simulink model "RefModel_GroundStation_FlightData"  (R2020b)
settings: Solver=FixedStepAuto  StartTime=0.0  StopTime=150  FixedStep=SimParam.GroundStation.Ts_base  RelTol=1e-3
values from neighbouring files (symbols this model uses):
  TASK_PARAM_V1000 = Simulink.Bus.createMATLABStruct('BUS_TASK_PATH_AlgoParam')    [INIT_Task.m]    (also in INIT_TaskManage.m)
undefined symbols (not defined in the file or in its folder): count, distBack, distFront, distLeft, distRight, ENUM_FlightTaskMode, flightTaskMode, groundspeedCmd, headingCmd, heightCmd, isRemoteConnected, isStationConnected, maxClimbSpeed, nBack, nFront, nLeft, nRight, param1_lond, param1_pointNumber, param2_latd, param3_relativeHeight, param4_radius, SimParam, stationLostTimeSec, unlock
settings Model: PauseTimes=0  Creator=sl  LastModifiedBy=sl
settings DataIOCC: SaveOutput=off  SaveTime=off  ReturnWorkspaceOutputs=off
settings DebuggingCC: InheritedTsInSrcMsg=none  UnderSpecifiedDimensionMsg=warning  ArithmeticOperatorsInVariantConditions=warning
settings SFSimCC: CustomCodeUndefinedFunction=UseInterfaceOnly
settings GRTTargetCC: CombineOutputUpdateFcns=off  MatFileLogging=off

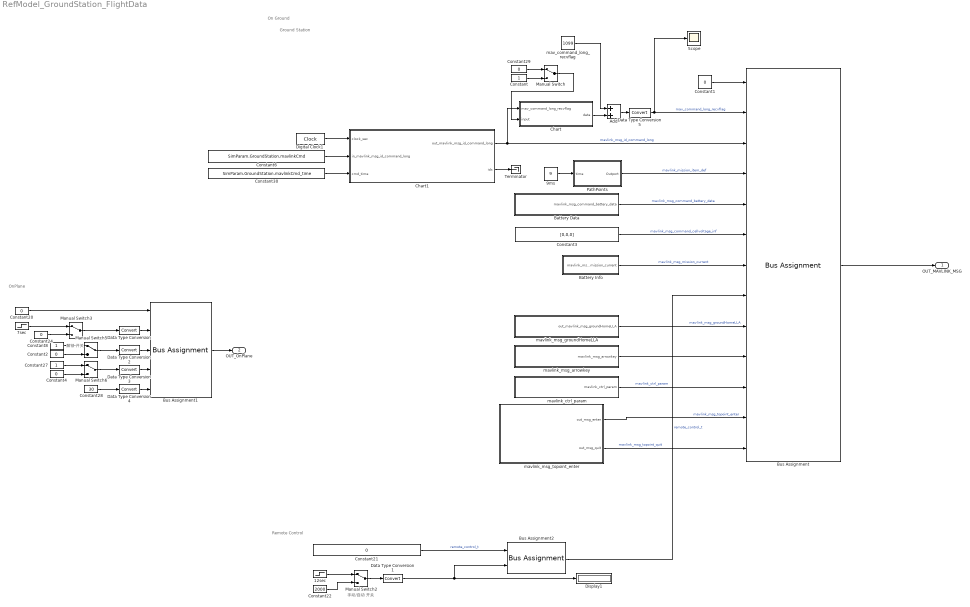
== system RefModel_GroundStation_FlightData ==
  note: 手动/自动 开关
  note: Ground Station
  note: Remote Control
  note: OnPlane
  note: On Ground
  note: 解锁 开关
  12sec : Step  Time=12+30  Before=2000  After=1000  SampleTime=SimParam.GroundStation.Ts_base  mask(DiscretizedSource){}
      mask init:
      | %zoh
  7sec : Step  Time=7+30  SampleTime=SimParam.GroundStation.Ts_base  mask(DiscretizedSource){}
      mask init:
      | %zoh
  9ms : Constant  Value=9
  Add : Sum
  Battery Data : Subsystem
  Battery Info : Subsystem
  Bus Assignment : BusAssignment  AssignedSignals=mav_command_long_recvflag,mavlink_msg_id_command_long,mavlink_mission_item_def,mavlink_msg_command_battery_data,mavlink_msg_command_cellvoltage_inf,mavlink_msg_mission_current,remote_control_t,mavlink_msg_groundHomeLLA,mavlink_msg_arrowkey,mavlink_ctrl_param,mavlink_msg_topoint_enter,mavlink_msg_topoint_quit
  Bus Assignment1 : BusAssignment  AssignedSignals=unlock,isRemoteConnected,isStationConnected,stationLostTimeSec
  Bus Assignment2 : BusAssignment  AssignedSignals=chG_Mag
  Chart : Stateflow chart  TreatAsAtomicUnit=on
  Chart1 : Stateflow chart  TreatAsAtomicUnit=on
  Constant : Constant
  Constant1 : Constant  Value=0  OutDataTypeStr=Bus: BUS_MAVLINK_TO_FIRM
  Constant{2,4,24,29} (4 alike) : Constant  Value=0
  Constant20 : Constant  Value=0  OutDataTypeStr=Bus: BUS_ONPLANE_FEEDBACK
  Constant21 : Constant  Value=0  OutDataTypeStr=Bus: remote_control_t
  Constant22 : Constant  Value=2000
  Constant27 : Constant
  Constant28 : Constant  Value=30
  Constant3 : Constant  Value=[0,0,0]  OutDataTypeStr=Bus: mavlink_msg_command_cellvoltage_inf
  Constant30 : Constant  Value=SimParam.GroundStation.mavlinkCmd_time
  Constant6 : Constant  Value=SimParam.GroundStation.mavlinkCmd  OutDataTypeStr=Bus: mavlink_msg_id_command_long
  Constant8 : Constant
  Data Type Conversion{,1..5} (6 alike) : DataTypeConversion
  Digital Clock1 : DigitalClock  SampleTime=-1
  Display1 : Display
  Manual Switch{,2..3,5..6} (5 alike) : ManualSwitch
  PathPoints : Subsystem
  Scope : Scope
  Terminator : Terminator
  mav_command_long_recvflag : Constant  Value=1099
  mavlink_ctrl_param : Subsystem
  mavlink_msg_arrowkey : Subsystem
  mavlink_msg_groundHomeLLA : Subsystem
  mavlink_msg_topoint_enter : Subsystem
  OUT_MAVLINK_MSG : Outport  OutDataTypeStr=Bus: BUS_MAVLINK_TO_FIRM  BusOutputAsStruct=on
  OUT_OnPlane : Outport  Port=2  OutDataTypeStr=Bus: BUS_ONPLANE_FEEDBACK
  wires:
  Bus Assignment/1 -> OUT_MAVLINK_MSG/1
  Bus Assignment1/1 -> OUT_OnPlane/1
  Battery Info/1(mavlink_msg_mission_current) -> Bus Assignment/7  "mavlink_msg_mission_current"
  Constant3/1 -> Bus Assignment/6  "mavlink_msg_command_cellvoltage_inf"
  PathPoints/1(Outport) -> Bus Assignment/4  "mavlink_mission_item_def"
  Chart1/1(out_mavlink_msg_id_command_long) -> Bus Assignment/3, Chart/1(mav_command_long_recvflag)  "mavlink_msg_id_command_long"
  Constant20/1 -> Bus Assignment1/1
  Constant21/1 -> Bus Assignment2/1  "remote_control_t"
  Bus Assignment2/1 -> Bus Assignment/8  "remote_control_t"
  Data Type Conversion1/1 -> Bus Assignment2/2, Display1/1
  Manual Switch2/1 -> Data Type Conversion1/1
  12sec/1 -> Manual Switch2/1
  Constant22/1 -> Manual Switch2/2
  Constant24/1 -> Manual Switch3/2
  Data Type Conversion/1 -> Bus Assignment1/2
  7sec/1 -> Manual Switch3/1
  Manual Switch3/1 -> Data Type Conversion/1
  Battery Data/1(mavlink_msg_command_battery_data) -> Bus Assignment/5  "mavlink_msg_command_battery_data"
  Data Type Conversion2/1 -> Bus Assignment1/3
  Data Type Conversion3/1 -> Bus Assignment1/4
  Data Type Conversion4/1 -> Bus Assignment1/5
  Constant28/1 -> Data Type Conversion4/1
  Manual Switch5/1 -> Data Type Conversion2/1
  Constant8/1 -> Manual Switch5/1
  Constant2/1 -> Manual Switch5/2
  Constant4/1 -> Manual Switch6/2
  Constant27/1 -> Manual Switch6/1
  Manual Switch6/1 -> Data Type Conversion3/1
  9ms/1 -> PathPoints/1(time)
  Constant29/1 -> Manual Switch/1
  Constant/1 -> Manual Switch/2
  Manual Switch/1 -> Chart/2(input)
  Data Type Conversion5/1 -> Bus Assignment/2, Scope/1  "mav_command_long_recvflag"
  mavlink_msg_groundHomeLLA/1(out_mavlink_msg_groundHomeLLA) -> Bus Assignment/9  "mavlink_msg_groundHomeLLA"
  Chart/1(data) -> Add/2
  Add/1 -> Data Type Conversion5/1
  mav_command_long_recvflag/1 -> Add/1
  mavlink_msg_arrowkey/1(mavlink_msg_arrowkey) -> Bus Assignment/10
  mavlink_ctrl_param/1(mavlink_ctrl_param) -> Bus Assignment/11  "mavlink_ctrl_param"
  Constant30/1 -> Chart1/3(cmd_time)
  Digital Clock1/1 -> Chart1/1(clock_sec)
  Constant6/1 -> Chart1/2(in_mavlink_msg_id_command_long)
  Chart1/2(idx) -> Terminator/1
  mavlink_msg_topoint_enter/2(out_msg_quit) -> Bus Assignment/13  "mavlink_msg_topoint_quit"
  mavlink_msg_topoint_enter/1(out_msg_enter) -> Bus Assignment/12  "mavlink_msg_topoint_enter"
  Constant1/1 -> Bus Assignment/1

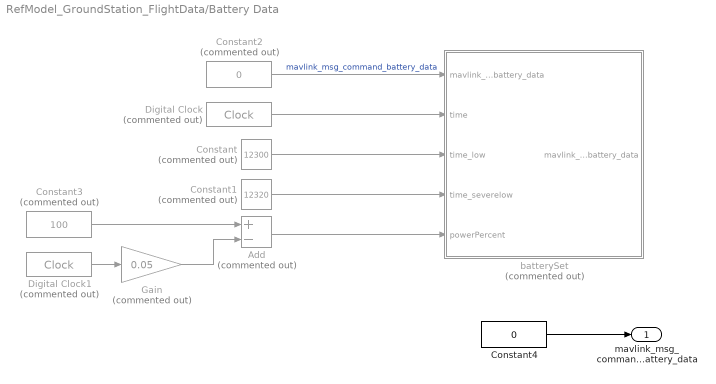
== system RefModel_GroundStation_FlightData/Battery Data ==
  Add : Sum  Commented=on  Inputs=+-
  Constant : Constant  Commented=on  Value=12300
  Constant1 : Constant  Commented=on  Value=12320
  Constant2 : Constant  Commented=on  Value=0  OutDataTypeStr=Bus: mavlink_msg_command_battery_data
  Constant3 : Constant  Commented=on  Value=100
  Constant4 : Constant  Value=0  OutDataTypeStr=Bus: mavlink_msg_command_battery_data
  Digital Clock : DigitalClock  Commented=on  SampleTime=-1
  Digital Clock1 : DigitalClock  Commented=on  SampleTime=-1
  Gain : Gain  Commented=on  Gain=0.05
  batterySet : MATLAB Function  Commented=on  TreatAsAtomicUnit=on
  mavlink_msg_command_battery_data : Outport
  wires:
  Constant2/1 -> batterySet/1("mavlink_msg_command_battery_data ")  "mavlink_msg_command_battery_data"
  Constant4/1 -> mavlink_msg_command_battery_data/1
  Digital Clock/1 -> batterySet/2(time)
  Constant/1 -> batterySet/3(time_low)
  Constant1/1 -> batterySet/4(time_severelow)
  Add/1 -> batterySet/5(powerPercent)
  Constant3/1 -> Add/1
  Digital Clock1/1 -> Gain/1
  Gain/1 -> Add/2

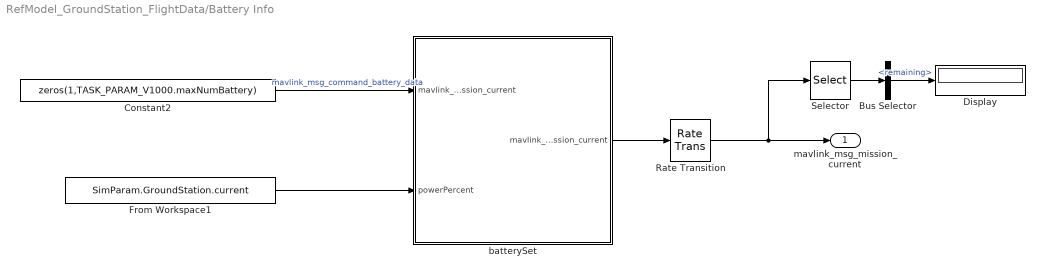
== system RefModel_GroundStation_FlightData/Battery Info ==
  Bus Selector : BusSelector  OutputSignals=remaining
  Constant2 : Constant  Value=zeros(1,TASK_PARAM_V1000.maxNumBattery)  OutDataTypeStr=Bus: mavlink_msg_mission_current
  Display : Display
  From Workspace1 : FromWorkspace  VariableName=SimParam.GroundStation.current  OutputAfterFinalValue=Holding final value
  Rate Transition : RateTransition
  Selector : Selector  InputPortWidth=TASK_PARAM_V1000.maxNumBattery  IndexOptions=Index vector (dialog)  Indices=1  OutputSizes=1
  batterySet : MATLAB Function  TreatAsAtomicUnit=on
  mavlink_msg_mission_current : Outport
  wires:
  From Workspace1/1 -> batterySet/2(powerPercent)
  batterySet/1(mavlink_msg_mission_current) -> Rate Transition/1
  Constant2/1 -> batterySet/1("mavlink_msg_mission_current ")  "mavlink_msg_command_battery_data"
  Rate Transition/1 -> Selector/1, mavlink_msg_mission_current/1
  Selector/1 -> Bus Selector/1
  Bus Selector/1 -> Display/1  "<remaining>"

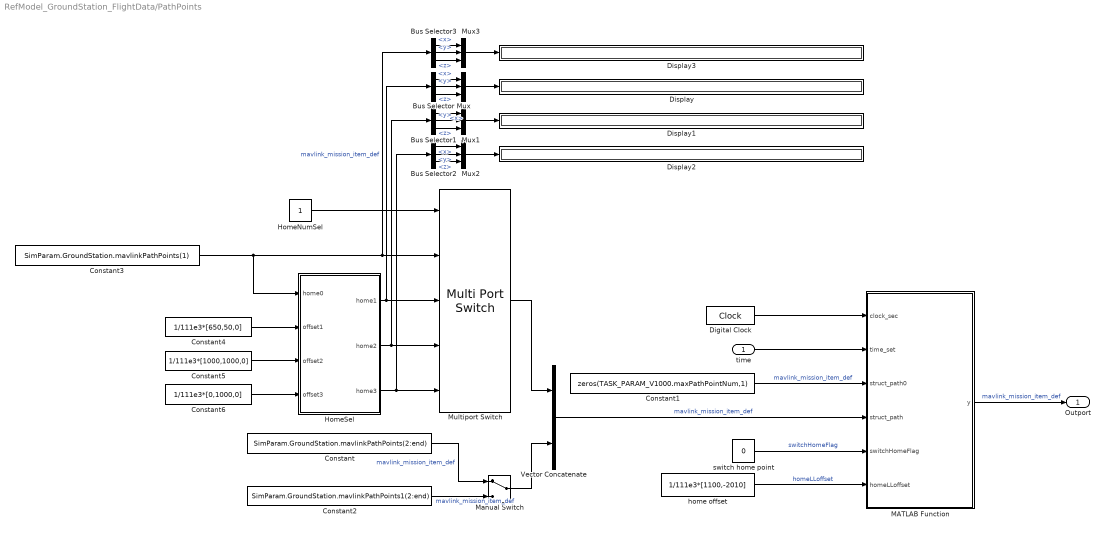
== system RefModel_GroundStation_FlightData/PathPoints ==
  time : Inport
  Bus Selector{,1..3} (4 alike) : BusSelector  OutputSignals=x,y,z
  Constant : Constant  Value=SimParam.GroundStation.mavlinkPathPoints(2:end)  OutDataTypeStr=Bus: mavlink_mission_item_def
  Constant1 : Constant  Value=zeros(TASK_PARAM_V1000.maxPathPointNum,1)  OutDataTypeStr=Bus: mavlink_mission_item_def
  Constant2 : Constant  Value=SimParam.GroundStation.mavlinkPathPoints1(2:end)  OutDataTypeStr=Bus: mavlink_mission_item_def
  Constant3 : Constant  Value=SimParam.GroundStation.mavlinkPathPoints(1)  OutDataTypeStr=Bus: mavlink_mission_item_def
  Constant4 : Constant  Value=1/111e3*[650,50,0]
  Constant5 : Constant  Value=1/111e3*[1000,1000,0]
  Constant6 : Constant  Value=1/111e3*[0,1000,0]
  Digital Clock : DigitalClock  SampleTime=-1
  Display{,1..3} (4 alike) : Display
  HomeNumSel : Constant
  HomeSel : MATLAB Function  TreatAsAtomicUnit=on
  MATLAB Function : MATLAB Function  TreatAsAtomicUnit=on
  Manual Switch : ManualSwitch
  Multiport Switch : MultiPortSwitch  Inputs=4
  Mux{,1..3} (4 alike) : Mux  Inputs=3
  Vector Concatenate : Concatenate
  home offset : Constant  Value=1/111e3*[1100,-2010]
  switch home point : Constant  Value=0
  Outport : Outport
  wires:
  MATLAB Function/1(y) -> Outport/1  "mavlink_mission_item_def"
  Digital Clock/1 -> MATLAB Function/1(clock_sec)
  time/1 -> MATLAB Function/2(time_set)
  Constant1/1 -> MATLAB Function/3(struct_path0)  "mavlink_mission_item_def"
  Vector Concatenate/1 -> MATLAB Function/4(struct_path)  "mavlink_mission_item_def"
  switch home point/1 -> MATLAB Function/5(switchHomeFlag)  "switchHomeFlag"
  home offset/1 -> MATLAB Function/6(homeLLoffset)  "homeLLoffset"
  Constant/1 -> Manual Switch/1  "mavlink_mission_item_def"
  HomeNumSel/1 -> Multiport Switch/1
  Multiport Switch/1 -> Vector Concatenate/1
  Constant3/1 -> HomeSel/1(home0), Bus Selector3/1, Multiport Switch/2  "mavlink_mission_item_def"
  Constant4/1 -> HomeSel/2(offset1)
  Constant5/1 -> HomeSel/3(offset2)
  Constant6/1 -> HomeSel/4(offset3)
  HomeSel/3(home3) -> Bus Selector2/1, Multiport Switch/5
  HomeSel/2(home2) -> Bus Selector1/1, Multiport Switch/4
  HomeSel/1(home1) -> Bus Selector/1, Multiport Switch/3
  Bus Selector/1 -> Mux/1  "<x>"
  Bus Selector/2 -> Mux/2  "<y>"
  Bus Selector/3 -> Mux/3  "<z>"
  Mux/1 -> Display/1
  Mux1/1 -> Display1/1
  Bus Selector1/3 -> Mux1/3  "<z>"
  Bus Selector1/2 -> Mux1/2  "<y>"
  Bus Selector1/1 -> Mux1/1  "<x>"
  Bus Selector2/1 -> Mux2/1  "<x>"
  Bus Selector2/2 -> Mux2/2  "<y>"
  Bus Selector2/3 -> Mux2/3  "<z>"
  Mux2/1 -> Display2/1
  Mux3/1 -> Display3/1
  Bus Selector3/3 -> Mux3/3  "<z>"
  Bus Selector3/2 -> Mux3/2  "<y>"
  Bus Selector3/1 -> Mux3/1  "<x>"
  Constant2/1 -> Manual Switch/2  "mavlink_mission_item_def"
  Manual Switch/1 -> Vector Concatenate/2

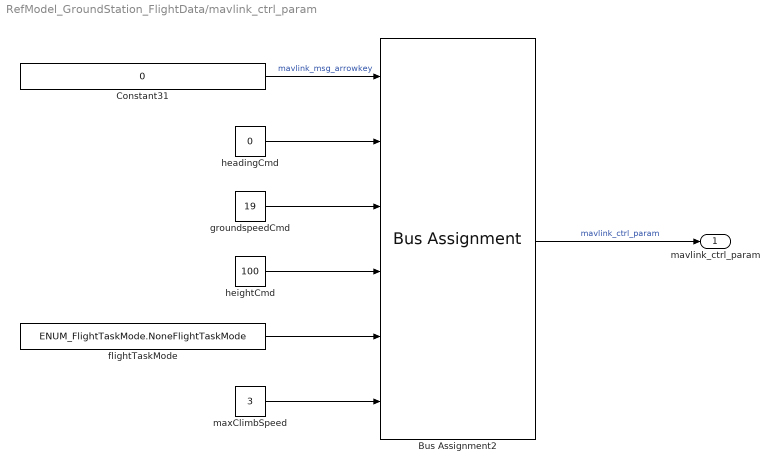
== system RefModel_GroundStation_FlightData/mavlink_ctrl_param ==
  Bus Assignment2 : BusAssignment  AssignedSignals=headingCmd,groundspeedCmd,heightCmd,flightTaskMode,maxClimbSpeed
  Constant31 : Constant  Value=0  OutDataTypeStr=Bus: mavlink_ctrl_param
  flightTaskMode : Constant  Value=ENUM_FlightTaskMode.NoneFlightTaskMode
  groundspeedCmd : Constant  Value=19
  headingCmd : Constant  Value=0
  heightCmd : Constant  Value=100
  maxClimbSpeed : Constant  Value=3
  mavlink_ctrl_param : Outport
  wires:
  Constant31/1 -> Bus Assignment2/1  "mavlink_msg_arrowkey"
  Bus Assignment2/1 -> mavlink_ctrl_param/1  "mavlink_ctrl_param"
  headingCmd/1 -> Bus Assignment2/2
  groundspeedCmd/1 -> Bus Assignment2/3
  heightCmd/1 -> Bus Assignment2/4
  maxClimbSpeed/1 -> Bus Assignment2/6
  flightTaskMode/1 -> Bus Assignment2/5

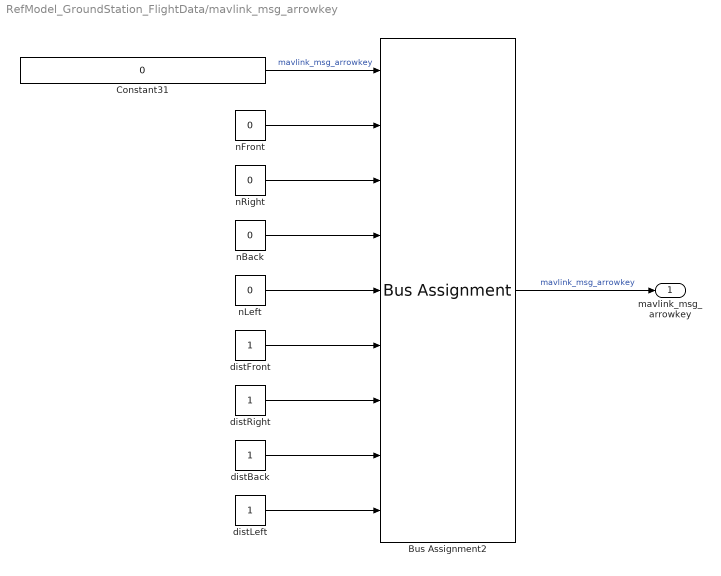
== system RefModel_GroundStation_FlightData/mavlink_msg_arrowkey ==
  Bus Assignment2 : BusAssignment  AssignedSignals=nFront,nRight,nBack,nLeft,distFront,distRight,distBack,distLeft
  Constant31 : Constant  Value=0  OutDataTypeStr=Bus: BUS_TASK_ARROWKEY
  distBack : Constant
  distFront : Constant
  distLeft : Constant
  distRight : Constant
  nBack : Constant  Value=0
  nFront : Constant  Value=0
  nLeft : Constant  Value=0
  nRight : Constant  Value=0
  mavlink_msg_arrowkey : Outport
  wires:
  Bus Assignment2/1 -> mavlink_msg_arrowkey/1  "mavlink_msg_arrowkey"
  Constant31/1 -> Bus Assignment2/1  "mavlink_msg_arrowkey"
  nFront/1 -> Bus Assignment2/2
  nRight/1 -> Bus Assignment2/3
  nBack/1 -> Bus Assignment2/4
  nLeft/1 -> Bus Assignment2/5
  distFront/1 -> Bus Assignment2/6
  distRight/1 -> Bus Assignment2/7
  distBack/1 -> Bus Assignment2/8
  distLeft/1 -> Bus Assignment2/9

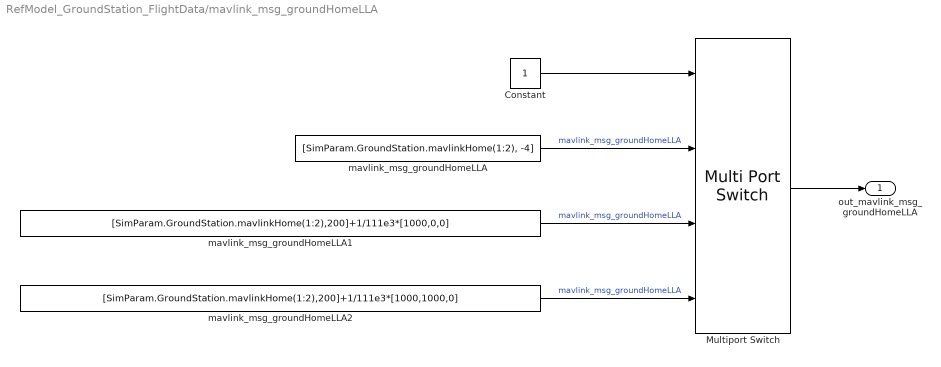
== system RefModel_GroundStation_FlightData/mavlink_msg_groundHomeLLA ==
  Constant : Constant
  Multiport Switch : MultiPortSwitch
  mavlink_msg_groundHomeLLA : Constant  Value=[SimParam.GroundStation.mavlinkHome(1:2), -4]  OutDataTypeStr=Inherit: Inherit via back propagation
  mavlink_msg_groundHomeLLA1 : Constant  Value=[SimParam.GroundStation.mavlinkHome(1:2),200]+1/111e3*[1000,0,0]  OutDataTypeStr=Inherit: Inherit via back propagation
  mavlink_msg_groundHomeLLA2 : Constant  Value=[SimParam.GroundStation.mavlinkHome(1:2),200]+1/111e3*[1000,1000,0]  OutDataTypeStr=Inherit: Inherit via back propagation
  out_mavlink_msg_groundHomeLLA : Outport
  wires:
  mavlink_msg_groundHomeLLA/1 -> Multiport Switch/2  "mavlink_msg_groundHomeLLA"
  Multiport Switch/1 -> out_mavlink_msg_groundHomeLLA/1
  Constant/1 -> Multiport Switch/1
  mavlink_msg_groundHomeLLA1/1 -> Multiport Switch/3  "mavlink_msg_groundHomeLLA"
  mavlink_msg_groundHomeLLA2/1 -> Multiport Switch/4  "mavlink_msg_groundHomeLLA"

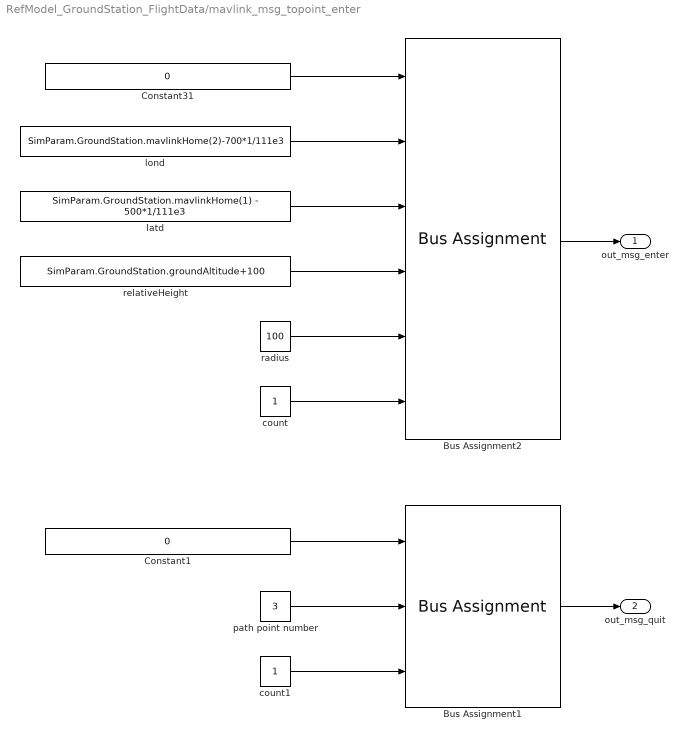
== system RefModel_GroundStation_FlightData/mavlink_msg_topoint_enter ==
  Bus Assignment1 : BusAssignment  AssignedSignals=param1_pointNumber,count
  Bus Assignment2 : BusAssignment  AssignedSignals=param1_lond,param2_latd,param3_relativeHeight,param4_radius,count
  Constant1 : Constant  Value=0  OutDataTypeStr=Bus: BUS_MAVLINK_ToPointAndHover_Quit
  Constant31 : Constant  Value=0  OutDataTypeStr=Bus: BUS_MAVLINK_ToPointAndHover_Enter
  count : Constant
  count1 : Constant
  latd : Constant  Value=SimParam.GroundStation.mavlinkHome(1) - 500*1/111e3
  lond : Constant  Value=SimParam.GroundStation.mavlinkHome(2)-700*1/111e3
  path point number : Constant  Value=3
  radius : Constant  Value=100
  relativeHeight : Constant  Value=SimParam.GroundStation.groundAltitude+100
  out_msg_enter : Outport
  out_msg_quit : Outport  Port=2
  wires:
  radius/1 -> Bus Assignment2/5
  count/1 -> Bus Assignment2/6
  relativeHeight/1 -> Bus Assignment2/4
  latd/1 -> Bus Assignment2/3
  lond/1 -> Bus Assignment2/2
  Bus Assignment2/1 -> out_msg_enter/1
  Constant31/1 -> Bus Assignment2/1
  Bus Assignment1/1 -> out_msg_quit/1
  path point number/1 -> Bus Assignment1/2
  Constant1/1 -> Bus Assignment1/1
  count1/1 -> Bus Assignment1/3

== matlab function RefModel_GroundStation_FlightData/Battery Data/batterySet ==
  data: mavlink_msg_command_battery_data input Bus: mavlink_msg_command_battery_data; mavlink_msg_command_battery_data output size=3; time input; time_low input; time_severelow input; powerPercent input
function mavlink_msg_command_battery_data  = fcn(mavlink_msg_command_battery_data, time, time_low, time_severelow,powerPercent)
if time > time_low && time <= time_severelow
    mavlink_msg_command_battery_data.battery(1).lifePercent = uint8(19);
    mavlink_msg_command_battery_data.battery(2).lifePercent = uint8(20);
    mavlink_msg_command_battery_data.battery(3).lifePercent = uint8(22);
elseif time > time_severelow
    mavlink_msg_command_battery_data.battery(1).lifePercent = uint8(6);
    mavlink_msg_command_battery_data.battery(2).lifePercent = uint8(4);
    mavlink_msg_command_battery_data.battery(3).lifePercent = uint8(6);
elseif time < 10
    mavlink_msg_command_battery_data.battery(1).lifePercent = uint8(0);
    mavlink_msg_command_battery_data.battery(2).lifePercent = uint8(0);
    mavlink_msg_command_battery_data.battery(3).lifePercent = uint8(0);
else
    mavlink_msg_command_battery_data.battery(1).lifePercent = uint8(powerPercent);
    mavlink_msg_command_battery_data.battery(2).lifePercent = uint8(powerPercent);
    mavlink_msg_command_battery_data.battery(3).lifePercent = uint8(powerPercent);
end

== matlab function RefModel_GroundStation_FlightData/PathPoints/MATLAB Function ==
  data: clock_sec input; y output Bus: mavlink_mission_item_def; time_set input; struct_path0 input Bus: mavlink_mission_item_def; struct_path input Bus: mavlink_mission_item_def; switchHomeFlag input; homeLLoffset input
function y = fcn(clock_sec,time_set,struct_path0,struct_path, switchHomeFlag, homeLLoffset)
if clock_sec > time_set 
    y = struct_path;
    if switchHomeFlag
        y(1).x = y(1).x + homeLLoffset(1);
        y(1).y = y(1).y + homeLLoffset(2);
    end
else
    y = struct_path0;
end

== stateflow chart RefModel_GroundStation_FlightData/Chart ==
  state State
    en:
    data = 0;
    du:
    data = data + input;
    if hasChanged(mav_command_long_recvflag.command)
    data = data + 1;
    end
  (default) -> State
  data: mav_command_long_recvflag input; data output; input input

== matlab function RefModel_GroundStation_FlightData/Battery Info/batterySet ==
  data: mavlink_msg_mission_current input Bus: mavlink_msg_mission_current; mavlink_msg_mission_current output size=3; powerPercent input
function mavlink_msg_mission_current  = fcn(mavlink_msg_mission_current,powerPercent)
mavlink_msg_mission_current(1).remaining = int8(powerPercent);
mavlink_msg_mission_current(2).remaining = int8(powerPercent);
mavlink_msg_mission_current(3).remaining = int8(powerPercent);

% mavlink_msg_mission_current(1).remaining = int8(0);
% mavlink_msg_mission_current(2).remaining = int8(0);
% mavlink_msg_mission_current(3).remaining = int8(0);

== matlab function RefModel_GroundStation_FlightData/PathPoints/HomeSel ==
  data: home0 input Bus: mavlink_mission_item_def; home1 output Bus: mavlink_mission_item_def; offset1 input; offset2 input; home2 output Bus: mavlink_mission_item_def; offset3 input; home3 output Bus: mavlink_mission_item_def
function [home1,home2,home3] = fcn(home0, offset1, offset2, offset3)
home1 = home0;
home1.x = home0.x + offset1(1);
home1.y = home0.y + offset1(2);
home2 = home0;
home2.x = home0.x + offset2(1);
home2.y = home0.y + offset2(2);
home3 = home0;
home3.x = home0.x + offset3(1);
home3.y = home0.y + offset3(2);

== stateflow chart RefModel_GroundStation_FlightData/Chart1 ==
  state Before
    en:
  state Doing
    en:
    idx = idx + 1;
    if in_mavlink_msg_id_command_long(idx).command ~= 0
    out_mavlink_msg_id_command_long = in_mavlink_msg_id_command_long(idx);
    end
    du:
  state After
    en:
    idx = idx + 1;
    if in_mavlink_msg_id_command_long(idx).command ~= 0
    out_mavlink_msg_id_command_long = in_mavlink_msg_id_command_long(idx);
    end
  (default) -> Before : {idx = 0;}
  Before -> Doing : [isOverFirstTime]
  (junction 20) -> Doing
  Doing -> (junction 15)
  (junction 15) -> (junction 20) [order 1] : [~isOverLastTime && isAllowGoToNext]
  (junction 15) -> After [order 2] : [isOverLastTime]
  data: flag function_output; flag function_output; flag function_output; clock_sec input; in_mavlink_msg_id_command_long input Bus: mavlink_msg_id_command_long size=200; out_mavlink_msg_id_command_long output Bus: mavlink_msg_id_command_long size=1; cmd_time input; idx output
  function flag = isOverLastTime:
    | function flag = isOverLastTime
    | flag = false;
    | if cmd_time(idx) == 0
    |     flag = true; 
    | end
  function flag = isOverFirstTime:
    | function flag = isOverFirstTime
    | % 达到第一个时间
    | flag = false;
    | if clock_sec >= cmd_time(1)
    |     flag = true; 
    | end
  function flag = isAllowGoToNext:
    | function flag = isAllowGoToNext
    | if idx < length(cmd_time) && ... % 索引保护
    |         cmd_time(idx+1) ~= 0     % 下一位为有效值
    |     time_threshold = cmd_time(idx+1);
    | else
    |     time_threshold = inf;
    | end
    | 
    | flag = false;
    | if clock_sec >= cmd_time(idx+1) && ...
    |         in_mavlink_msg_id_command_long(idx).command ~= 0
    |     flag = true; 
    | end
